simulink model "model_dyskretna_transmitancja"  (R2023b)
settings: Solver=FixedStepDiscrete  StartTime=0.0  StopTime=5000  FixedStep=10  RelTol=1e-3
settings Model: Creator=tototmek  LastModifiedBy=tototmek

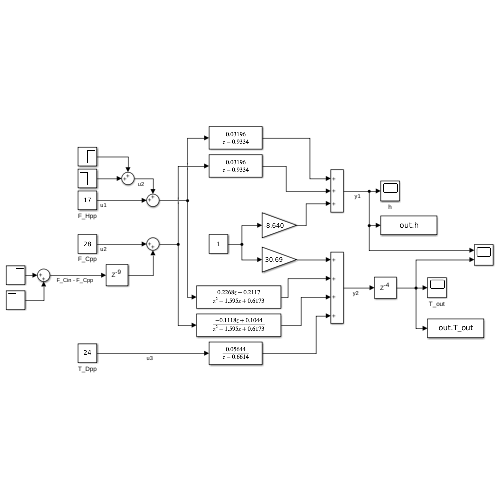
[thumbnail: Simulink's stored preview of the top-level diagram]
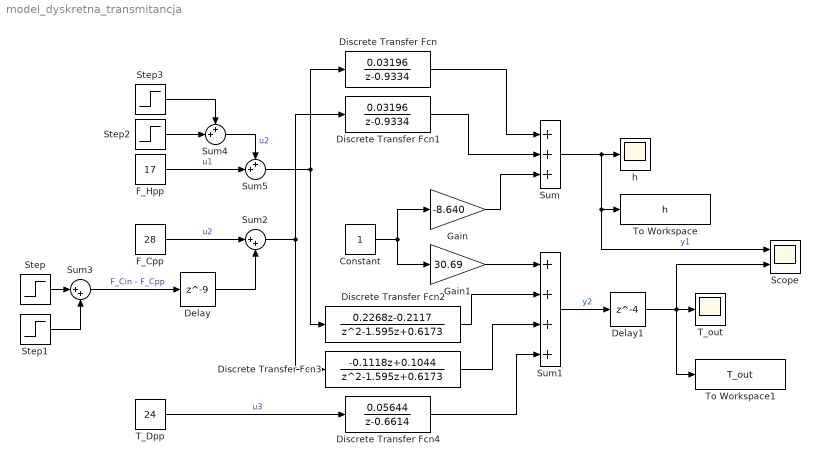
== system model_dyskretna_transmitancja ==
  Constant : Constant
  Delay : Delay  DelayLength=9
  Delay1 : Delay  DelayLength=4  InitialCondition=36.83333333
  Discrete Transfer Fcn : DiscreteTransferFcn  Numerator=[0.03196]  Denominator=[1 -0.9334]
  Discrete Transfer Fcn1 : DiscreteTransferFcn  Numerator=[0.03196]  Denominator=[1 -0.9334]
  Discrete Transfer Fcn2 : DiscreteTransferFcn  Numerator=[0.2268 -0.2117]  Denominator=[1 -1.595 0.6173]
  Discrete Transfer Fcn3 : DiscreteTransferFcn  Numerator=[-0.1118 0.1044]  Denominator=[1 -1.595 0.6173]
  Discrete Transfer Fcn4 : DiscreteTransferFcn  Numerator=[0.05644]  Denominator=[1 -0.6614]
  F_Cpp : Constant  Value=28
  F_Hpp : Constant  Value=17
  Gain : Gain  Gain=-8.640
  Gain1 : Gain  Gain=30.69
  Scope : Scope  NumInputPorts=2
  Step : Step  Time=2000  After=2.8  SampleTime=0
  Step1 : Step  Time=2500  After=-5.6  SampleTime=0
  Step2 : Step  Time=1500  After=-3.4  SampleTime=0
  Step3 : Step  Time=1000  After=1.7  SampleTime=0
  Sum : Sum  Inputs=+++
  Sum1 : Sum  Inputs=++++
  Sum2 : Sum  Inputs=|++
  Sum3 : Sum  Inputs=|++
  Sum4 : Sum  Inputs=++|
  Sum5 : Sum  Inputs=++|
  T_Dpp : Constant  Value=24
  T_out : Scope
  To Workspace : ToWorkspace  VariableName=h  SaveFormat=Timeseries  SampleTime=-1
  To Workspace1 : ToWorkspace  VariableName=T_out  SaveFormat=Timeseries  SampleTime=-1
  h : Scope
  wires:
  Sum/1 -> Scope/1, To Workspace/1, h/1  "y1"
  Sum3/1 -> Delay/1  "F_Cin - F_Cpp"
  Step/1 -> Sum3/1
  T_Dpp/1 -> Discrete Transfer Fcn4/1  "u3"
  Gain/1 -> Sum/3
  Discrete Transfer Fcn4/1 -> Sum1/4
  Delay/1 -> Sum2/2
  Gain1/1 -> Sum1/1
  Sum5/1 -> Discrete Transfer Fcn2/1, Discrete Transfer Fcn/1
  F_Hpp/1 -> Sum5/2  "u1"
  Discrete Transfer Fcn/1 -> Sum/1
  Sum2/1 -> Discrete Transfer Fcn3/1, Discrete Transfer Fcn1/1
  Discrete Transfer Fcn3/1 -> Sum1/3
  Sum1/1 -> Delay1/1  "y2"
  Discrete Transfer Fcn2/1 -> Sum1/2
  Step1/1 -> Sum3/2
  Constant/1 -> Gain/1, Gain1/1
  Discrete Transfer Fcn1/1 -> Sum/2
  Step3/1 -> Sum4/1
  F_Cpp/1 -> Sum2/1  "u2"
  Step2/1 -> Sum4/2
  Delay1/1 -> To Workspace1/1, Scope/2, T_out/1
  Sum4/1 -> Sum5/1  "u2"
